simulink model "steady_state_analysis"  (R2015a)
settings: Solver=ode45  SolverMode=SingleTasking  StartTime=0.0  StopTime=0.1  RelTol=1e-3  AbsTol=1e-6
libraries: powerlib x8
Description:
  | Copyright 2008-2015 The MathWorks, Inc.
settings Model: FPTRunName=Active  CovSFcnEnable=off  ExtModeTrigMode=oneshot  ExtModeArmWhenConnect=off  ExtModeAutoUpdateStatusClock=off  Creator=MathWorks  LastModifiedBy=Student
settings DataIOCC: LimitDataPoints=off  SignalLoggingSaveFormat=ModelDataLogs  SignalLoggingName=sigsOut
settings OptimizationCC: BlockReduction=off  BooleanDataType=off  ExpressionDepthLimit=2147483647  InitFltsAndDblsToZero=on  EfficientMapNaN2IntZero=off
settings DebuggingCC: SaveWithParameterizedLinksMsg=none  UnderspecifiedInitializationDetection=Classic  MergeDetectMultiDrivingBlocksExec=none  CheckExecutionContextPreStartOutputMsg=on  CheckExecutionContextRuntimeOutputMsg=on  SignalResolutionControl=TryResolveAllWithWarning  MultiTaskDSMMsg=warning  MultiTaskCondExecSysMsg=none  FcnCallInpInsideContextMsg=UseLocalSettings  StateNameClashWarn=warning
settings HardwareCC: TargetUnknown=on
settings GRTTargetCC: TargetFcnLib=ansi_tfl_tmw.mat  CombineOutputUpdateFcns=off  GRTInterface=on

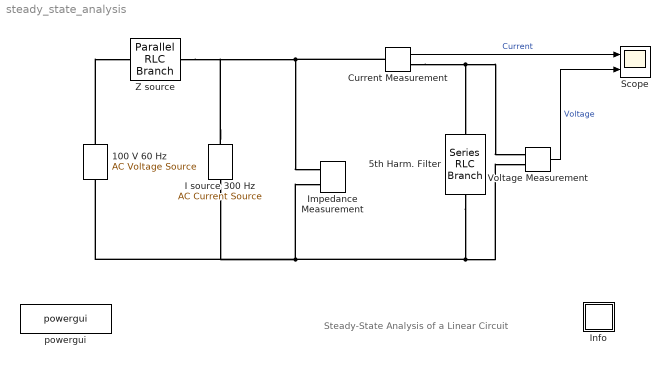
== system steady_state_analysis ==
  note: Steady-State Analysis of a Linear Circuit
  100 V 60 Hz : powerlib/Electrical Sources/AC Voltage Source  Description=source block  Amplitude=100  Phase=0  Frequency=60  SampleTime=0  Measurements=None
      settings: AttributesFormatString=\n
  5th Harm. Filter : powerlib/Elements/Series RLC Branch  LConnTagsString=__new0  RConnTagsString=__new0  BranchType=RLC  Resistance=1.27  Inductance=107.42e-03  SetiL0=off  InitialCurrent=0  Capacitance=2.62e-06  Setx0=off  InitialVoltage=0  Measurements=None
  Current Measurement : powerlib/Measurements/Current Measurement  Tag=PoWeRsYsTeMmEaSuReMeNt  PhasorSimulation=off  OutputType=Magnitude  PSBequivalent=0
  I source 300 Hz : powerlib/Electrical Sources/AC Current Source  Amplitude=10  Phase=-30  Frequency=300  SampleTime=0  Measurements=None
      settings: AttributesFormatString=\n
  Impedance Measurement : powerlib/Measurements/Impedance Measurement  LConnTagsString=+|-  Factor=1
      settings: AttributesFormatString=\n
  Info : Subsystem
      settings: OpenFcn=showdemo(bdroot(gcb))
      mask Display: disp('?')
  Scope : Scope  NumInputPorts=2
      settings: TimeRange=0.1  YMin=-10~-200  YMax=10~200
  Voltage Measurement : powerlib/Measurements/Voltage Measurement  Tag=PoWeRsYsTeMmEaSuReMeNt  PhasorSimulation=off  OutputType=Magnitude  PSBequivalent=0
  Z source : powerlib/Elements/Parallel RLC Branch  LConnTagsString=a  RConnTagsString=__new0  BranchType=RL  Resistance=37.7  Inductance=10e-03  SetiL0=off  InitialCurrent=0  Capacitance=0  Setx0=off  InitialVoltage=0  Measurements=None
  powergui : powerlib/powergui  Priority=2  SimulationMode=Continuous  SolverType=Tustin  SampleTime=50e-6  frequency=60  SPID=off  DisableSnubberDevices=off  DisableRonSwitches=off  DisableVfSwitches=off  SwTol=0  DisplayEquations=off  Interpol=off  methode=off  Ts=0  FunctionMessages=off  echomessages=off  HookPort=off  EnableUseOfTLC=off  x0status=blocks  frequencyindice=60  Pbase=100e6  ErrMax=1e-4  Iterations=50  UnitsV=kV  UnitsW=MW  buscounter=0  RestoreLinks=warning  ResistiveCurrentMeasurement=off  Frange=0:2:1000  Ylog=off  Xlog=off  ShowGrid=off  save=off  variable=ZData  structure=0  ZoomFFT=on  StartTime=0.0  cycles=1  DisplayStyle=off  fundamental=60  FreqAxis=off  MaxFrequency=1000  frequencyindicesteady=1  RmsSteady=1  display=off
  wires:
  Current Measurement/1 -> Scope/1  "Current"
  Voltage Measurement/1 -> Scope/2  "Voltage"
  connections:
  100 V 60 Hz/RConn1 -- Z source/LConn1
  Current Measurement/LConn1 -- I source 300 Hz/RConn1 -- Z source/RConn1 -- Impedance Measurement/LConn1
  5th Harm. Filter/RConn1 -- Impedance Measurement/LConn2 -- I source 300 Hz/LConn1 -- 100 V 60 Hz/LConn1 -- Voltage Measurement/LConn2
  Current Measurement/RConn1 -- 5th Harm. Filter/LConn1 -- Voltage Measurement/LConn1

== system steady_state_analysis/Info ==
